simulink model "ccmodel"  (R2017a)
settings: Solver=ode45  StartTime=0.0  StopTime=10.0  RelTol=1e-3
values from neighbouring files (symbols this model uses):
  b = 50    [setup_cruise_control.m]
  m = 1000    [setup_cruise_control.m]
undefined symbols (not defined in the file or in its folder): Ki, Kp
settings Model: Creator=sansh  LastModifiedBy=sansh

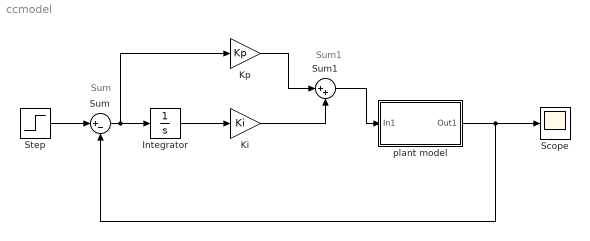
== system ccmodel ==
  note: Sum
  note: Sum1
  Integrator : Integrator
  Ki : Gain  Gain=Ki
  Kp : Gain  Gain=Kp
  Scope : Scope
  Step : Step  Time=0  After=u  SampleTime=0
  Sum : Sum  Inputs=|+-
  Sum1 : Sum  Inputs=|++
  plant model : Subsystem
  wires:
  plant model/1(Out1) -> Scope/1, Sum/2
  Sum/1 -> Kp/1, Integrator/1
  Integrator/1 -> Ki/1
  Sum1/1 -> plant model/1(In1)
  Ki/1 -> Sum1/2
  Kp/1 -> Sum1/1
  Step/1 -> Sum/1

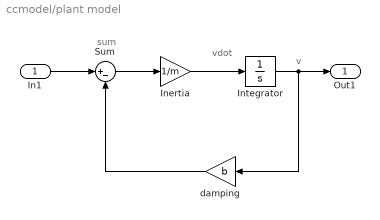
== system ccmodel/plant model ==
  note: vdot
  note: sum
  note: v
  In1 : Inport
  Inertia : Gain  Gain=1/m
  Integrator : Integrator
  Sum : Sum  Inputs=|+-
  damping : Gain  Gain=b
  Out1 : Outport
  wires:
  In1/1 -> Sum/1
  Sum/1 -> Inertia/1
  Inertia/1 -> Integrator/1
  damping/1 -> Sum/2
  Integrator/1 -> Out1/1, damping/1
